simulink model "V3_Modell"  (R2021a)
settings: Solver=ode3  StartTime=0.0  StopTime=Zeit(end)  FixedStep=0.001  RelTol=1e-3
values from neighbouring files (symbols this model uses):
  den = [L_A R_A]    [V3_Parameter.m]
  g = 9.81    [V3_Parameter.m]
  i_G = 62    [V3_Parameter.m]
  J = 5.5e-5 * i_G^2 + 0.003 + m_G * r_S^2    (= 0.23442)    [V3_Parameter.m]
  k_M = 0.106596822    [V3_Parameter.m]
  KL_REIB = [-2.355880331, -1.758035249, -1.164902556, -0.572712341, -0.001, 0, 0.001, 0.317929177, 0.917345055, 1.514352379, 2.115653213 ... (first row only)    [V3_Parameter.m]
  m_G = 2    [V3_Parameter.m]
  num = [1]    [V3_Parameter.m]
  r_S = 0.1    [V3_Parameter.m]
settings Model: Creator=schmi  LastModifiedBy=schmi

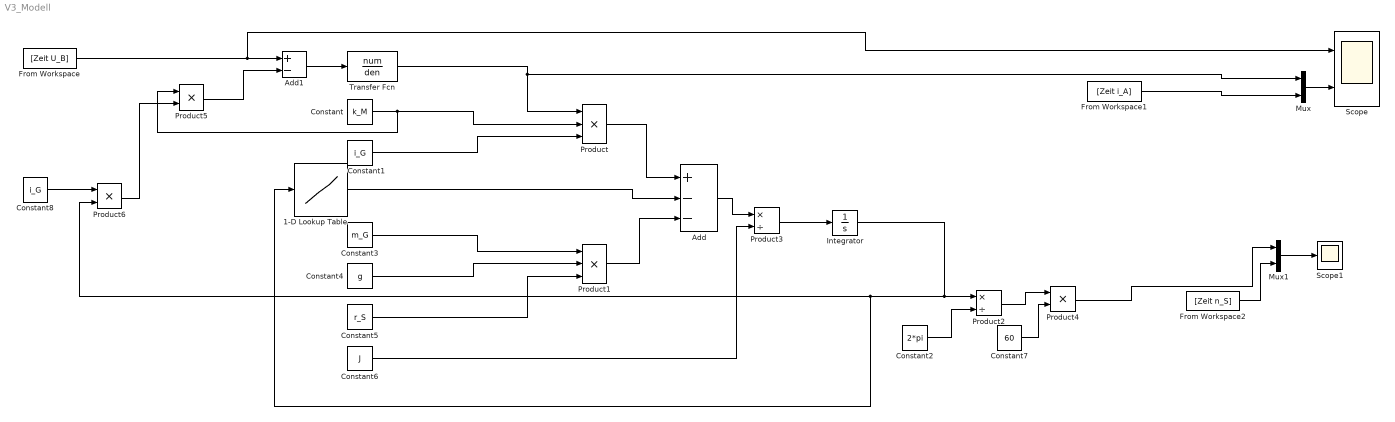
== system V3_Modell ==
  1-D Lookup Table : Lookup_n-D  NumberOfTableDimensions=1  BreakpointsForDimension1=KL_REIB(1,:)  Table=KL_REIB(2,:)  InternalRulePriority=Speed  RndMeth=Simplest  InputSameDT=on
  Add : Sum  Inputs=+--
  Add1 : Sum  Inputs=+-
  Constant : Constant  Value=k_M
  Constant1 : Constant  Value=i_G
  Constant2 : Constant  Value=2*pi
  Constant3 : Constant  Value=m_G
  Constant4 : Constant  Value=g
  Constant5 : Constant  Value=r_S
  Constant6 : Constant  Value=J
  Constant7 : Constant  Value=60
  Constant8 : Constant  Value=i_G
  From Workspace : FromWorkspace  VariableName=[Zeit U_B]
  From Workspace1 : FromWorkspace  VariableName=[Zeit i_A]
  From Workspace2 : FromWorkspace  VariableName=[Zeit n_S]
  Integrator : Integrator
  Mux : Mux  Inputs=2
  Mux1 : Mux  Inputs=2
  Product : Product  Inputs=3
  Product1 : Product  Inputs=3
  Product2 : Product  Inputs=*/
  Product3 : Product  Inputs=*/
  Product4 : Product
  Product5 : Product
  Product6 : Product
  Scope : Scope  NumInputPorts=2
  Scope1 : Scope
  Transfer Fcn : TransferFcn  Numerator=num  Denominator=den
  wires:
  Constant1/1 -> Product/3
  Constant/1 -> Product5/1, Product/2
  Transfer Fcn/1 -> Mux/1, Product/1
  Product/1 -> Add/1
  1-D Lookup Table/1 -> Add/2
  Constant3/1 -> Product1/1
  Constant4/1 -> Product1/2
  Constant5/1 -> Product1/3
  Product1/1 -> Add/3
  Product3/1 -> Integrator/1
  Add/1 -> Product3/1
  Integrator/1 -> Product6/2, 1-D Lookup Table/1, Product2/1
  Constant6/1 -> Product3/2
  Constant2/1 -> Product2/2
  Product2/1 -> Product4/1
  Constant7/1 -> Product4/2
  Product4/1 -> Mux1/1
  From Workspace/1 -> Scope/1, Add1/1
  Product5/1 -> Add1/2
  Add1/1 -> Transfer Fcn/1
  From Workspace1/1 -> Mux/2
  From Workspace2/1 -> Mux1/2
  Constant8/1 -> Product6/1
  Product6/1 -> Product5/2
  Mux/1 -> Scope/2
  Mux1/1 -> Scope1/1
